simulink model "analog_potentiometer"  (R2020b)
settings: Solver=ode1be  StartTime=0.0  StopTime=10  RelTol=1e-3  AbsTol=1e-3
libraries: analogCompBlocks x3, fl_lib x1, nesl_utility x1, ee_lib x1
settings Model: DataDictionary=analogComputerData.sldd  EnableAccessToBaseWorkspace=off  OrderedModelArguments=off  Creator=roadrunner  LastModifiedBy=roadrunner
settings SolverCC: AutoScaleAbsTol=off
settings DebuggingCC: SymbolicDimsDataTypeCodeGenerationDiagnostic=none
settings SFSimCC: CustomCodeUndefinedFunction=UseInterfaceOnly
settings SimscapeCC: SimscapeLogType=all  SimscapeLogSimulationStatistics=on  SimscapeLogDataHistory=10000

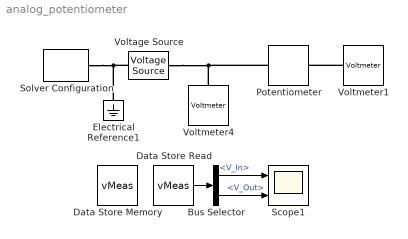
== system analog_potentiometer ==
  Bus Selector : BusSelector  OutputSignals=V_In,V_Out
  Data Store Memory : DataStoreMemory  Priority=5  DataStoreName=vMeas  ReadBeforeWriteMsg=warning  WriteAfterWriteMsg=warning  WriteAfterReadMsg=warning  ShowAdditionalParam=off  OutDataTypeStr=Bus: bus_const_multiplier_measurements
  Data Store Read : DataStoreRead  Priority=6  DataStoreName=vMeas
  Electrical Reference1 : fl_lib/Electrical/Electrical Elements/Electrical Reference
  Potentiometer : analogCompBlocks/Potentiometer  wiper_position=0.98  max_resistance=1  gain=10
      settings: AttributesFormatString=Potentiometer
  Scope1 : Scope  NumInputPorts=2
  Solver Configuration : nesl_utility/Solver Configuration  PhysicalDomain=network_engine_domain  SubClassName=solver  LeftPortType=input  RightPortType=generic  Tones=[]  Harmonics=[]  SimulateNoise=off  Profile=off  UseLocalSampling=off  EnableSwitchedLinearOptims=on  FrequencyDomain=off  UseCCode=off  RelTol=0.001  AbsTol=1e-06  MinStep=1e-09  ToWorkspace=off  RevertToSquareIcSolve=off  NumHomotopyIterations=100  PhasorMode=off  PhasorModeNumHarmonics=1  DoDC=off  ResidualTolerance=1e-09  UseLocalSolver=on  LocalSolverChoice=NE_BACKWARD_EULER_ADVANCER  LocalSolverSampleTime=0.01  DoFixedCost=on  MaxNonlinIter=3  MaxModeIter=2  ComputeImpulses=off  ImpulseIterations=2  LinearAlgebra=auto  EquationFormulation=NE_TIME_EF  DelaysMemoryBudget=1024  AutomaticFiltering=on  FilteringTimeConstant=0.001  PartitionStorageMethod=AS_NEEDED  PartitionMemoryBudget=1024  PartitionMethod=ROBUST
      settings: SourceProductName=Utilities
  Voltage Source : ee_lib/Sources/Voltage Source  dc_voltage=1 V  ac_voltage=0 V  ac_shift=0 rad  ac_frequency=60 Hz  noise_mode=0  PSD=0 V^2/Hz  repeatability=1  auto_seed=3538351120  user_seed=0  sample_time=1e-3 s  i_specify=off  i_priority=None  i=0 A  i_nominal_specify=off  i_nominal_unit=A  i_nominal_value=1  v_specify=off  v_priority=None  v=0 V  v_nominal_specify=off  v_nominal_unit=V  v_nominal_value=1
      settings: AttributesFormatString=Constant Voltage
  Voltmeter1 : analogCompBlocks/Voltmeter  Priority=4  DSNAME='vMeas'  DSELEMENT='V_Out'
      settings: AttributesFormatString=Voltage Sensor
  Voltmeter4 : analogCompBlocks/Voltmeter  Priority=2  DSNAME='vMeas'  DSELEMENT='V_In'
      settings: AttributesFormatString=Voltage Sensor
  wires:
  Data Store Read/1 -> Bus Selector/1
  Bus Selector/1 -> Scope1/1  "<V_In>"
  Bus Selector/2 -> Scope1/2  "<V_Out>"
  connections:
  Electrical Reference1/LConn1 -- Voltage Source/RConn1 -- Solver Configuration/RConn1
  Voltmeter4/LConn1 -- Potentiometer/LConn1 -- Voltage Source/LConn1
  Voltmeter1/LConn1 -- Potentiometer/RConn1
